simulink model "wheel_leg2"  (R2026a)
settings: Solver=VariableStepAuto  StopTime=7  MaxStep=0.01  AbsTol=1e-3  EnableMultiTasking=on
values from neighbouring files (symbols this model uses):
  K = lqr(A,B,Q,R)    [get_k_length.m]    (also in sys_lqr.m = sym('K',[2 6]))
  N = NM + mp*diff(x + L*sin(theta),t,2)    [get_k_length.m]
undefined symbols (not defined in the file or in its folder): X, Y, Z
libraries: sm_lib x87, nesl_utility x25, slpidlib x2
(part 1 of 3)
settings Model: Creator=86138  LastModifiedBy=Admin
settings SimscapeCC: SimscapeNominalValues="[{\"value\":\"1\",\"unit\":\"A\"},{\"value\":\"1\",\"unit\":\"bar\"},{\"value\":\"1\",\"unit\":\"cm^2\"},{\"value\":\"1\",\"unit\":\"cm^3/s\"},{\"value\":\"1\",\"unit\":\"kJ/kg\"},{\"value\":\"1\",\"unit\":\"kW\"},{\"value\":\"1\",\"unit\":\"l\"},{\"value\":\"1\",\"unit\":\"N\"},{\"value\":\"1\",\"unit\":\"N*m\"},{\"value\":\"1\",\"unit\":\"V\"}]"  SimscapeLogType=none  SimscapeLogSimulationStatistics=on
settings ExplorerConfigSet: InternalSimMechanicsExplorerSettings=|
  | <ExplorerConfiguration>
  | 
  |   <canonicalview>default</canonicalview>
  | 
  |   <TilePanel>
  |     <TileInfo>
  |       <Tiles Columns="1" Count="1" Height="898" Rows="1" Width="1720">
  |         <Row Weight="1"/>
  |         <Column Weight="1"/>
  |         <Tile Height="1" Width="1" X="0" Y="0"/>
  |       </Tiles>
  |     </TileInfo>
  |     <SceneInfo>
  |       <SceneViewer>
  |         <IsThisViewStd>
  |           <IsStandardView>off</IsStandardView>
  |           <StandardViewName>Front</StandardViewName>
  |         </IsThisViewStd>
  |         <BGColor>
  |           <R>0.85098039215686272</R>
  |           <G>0.85098039215686272</G>
  |           <B>0.85098039215686272</B>
  |           <A>1</A>
  |         </BGColor>
  |         <Camera>
  |           <DoPerspective>off</DoPerspective>
  |           <Position>
  |             <X>-61.687647663357318</X>
  |             <Y>-61.31400923411438</Y>
  |             <Z>24.215421272004388</Z>
  |           </Position>
  |           <Center>
  |             <X>-3.3890592997604467</X>
  |             <Y>3.6476545182531481</Y>
  |             <Z>2.021907302035288</Z>
  |           </Center>
  |           <Up>
  |             <X>0.16916832642928142</X>
  |             <Y>0.17928169149316647</Y>
  |             <Z>0.96914403079648859</Z>
  |           </Up>
  |           <XLim>2.9859335756375818</XLim>
  |           <YLim>2.9859335756375818</YLim>
  |           <ViewLimDist>0.01</ViewLimDist>
  |         </Camera>
  |       </SceneViewer>
  |     </SceneInfo>
  |   </TilePanel>
  | 
  |   <MechEditorPanel>
  |     <GfxPanelCameraMap/>
  |     <Cameras/>
  |     <VideoCreator>
  |       <IncludeTiles>All</IncludeTiles>
  |       <IncludeTime>on</IncludeTime>
  |       <IncludeWorldFrame>off</IncludeWorldFrame>
  |       <PlaybackSpeedRatio>0.5</PlaybackSpeedRatio>
  |       <FrameRate>30</FrameRate>
  |       <FrameSize>auto</FrameSize>
  |       <VideoFormat>MotionJPEGAVI</VideoFormat>
  |     </VideoCreator>
  |   </MechEditorPanel>
  | 
  |   <PlaybackSettings>
  |     <PlaybackSpeedFactor>0.5</PlaybackSpeedFactor>
  |   </PlaybackSettings>
  | 
  | </ExplorerConfiguration>

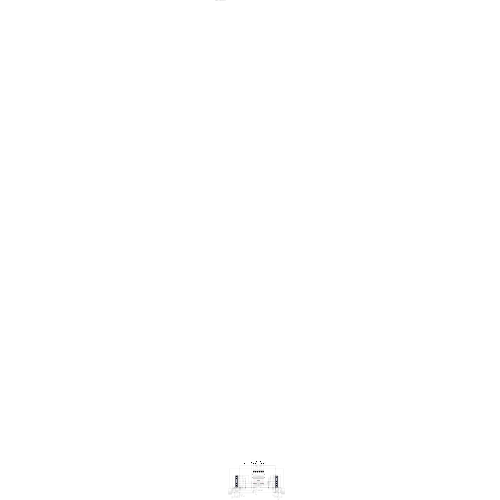
[thumbnail: Simulink's stored preview of the top-level diagram]
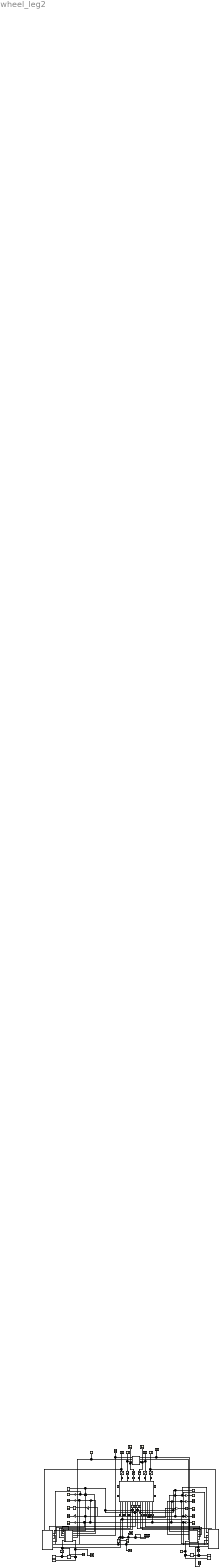
== system wheel_leg2 ==
  note: 参考开源文档作者：韭菜的菜 链接：https://zhuanlan.zhihu.com/p/613007726 来源：知乎
  note: K = get_k_length(0.25)
  Constant : Constant  Value=0.25
  Constant1 : Constant  Value=0.25
  Constant10 : Constant  Value=pi/2
  Constant12 : Constant  Value=pi/2
  Gain{22,24..26,33,36,38,40} (8 alike) : Gain  Gain=180/pi
  Gain29 : Gain  Gain=-0.06
  Gain41 : Gain  Gain=-0.06
  Integrator : Integrator
  Integrator2 : Integrator
  Integrator4 : Integrator
  L_X : Scope
      settings: ActiveDisplayYMinimum=-0.79846  ActiveDisplayYMaximum=7.01473
  L_d_phi : Scope
      settings: ActiveDisplayYMinimum=-7.35816  ActiveDisplayYMaximum=0.81757  DataLoggingVariableName=ScopeData2
  L_d_theta : Scope
      settings: ActiveDisplayYMinimum=-51.86845  ActiveDisplayYMaximum=175.83384  DataLoggingVariableName=ScopeData3
  L_phi : Scope
      settings: ActiveDisplayYMinimum=-1.27659  ActiveDisplayYMaximum=11.48927  DataLoggingVariableName=ScopeData4
  L_theta : Scope
      settings: ActiveDisplayYMinimum=-28.162  ActiveDisplayYMaximum=27.88738  DataLoggingVariableName=ScopeData5
  PID Controller2 : slpidlib/PID Controller  Controller=PID  Form=Parallel  TimeDomain=Continuous-time  UseExternalTs=off  SampleTime=-1  IntegratorMethod=Forward Euler  FilterMethod=Forward Euler  ControllerParametersSource=internal  P=500  I=0  UseKiTs=off  D=50  UseExternalDerivativeSource=off  N=100  UseFilter=on  TunerSelectOption=Transfer Function Based (PID Tuner App)  InitialConditionSource=internal  InitialConditionForIntegrator=0  InitialConditionForFilter=0  DifferentiatorICPrevScaledInput=0  ExternalReset=none  TrackingMode=off  Kt=1  LimitOutput=off  SatLimitsSource=internal  UpperSaturationLimit=inf  LowerSaturationLimit=-inf  LinearizeAsGain=on  AntiWindupMode=none  Kb=1  LimitIntegrator=off  UpperIntegratorSaturationLimit=inf  LowerIntegratorSaturationLimit=-inf  POutMin=[]  POutMax=[]  IOutMin=[]  IOutMax=[]  DOutMin=[]  DOutMax=[]  NOutMin=[]  NOutMax=[]  SumOutMin=[]  SumOutMax=[]  SaturationOutMin=[]  SaturationOutMax=[]  PParamMin=[]  PParamMax=[]  IParamMin=[]  IParamMax=[]  DParamMin=[]  DParamMax=[]  NParamMin=[]  NParamMax=[]  KbParamMin=[]  KbParamMax=[]  KtParamMin=[]  KtParamMax=[]  KbOutMin=[]  KbOutMax=[]  KtOutMin=[]  KtOutMax=[]  IntegratorOutMin=[]  IntegratorOutMax=[]  FilterOutMin=[]  FilterOutMax=[]  SumI1OutMin=[]  SumI1OutMax=[]  SumI2OutMin=[]  SumI2OutMax=[]  SumI3OutMin=[]  SumI3OutMax=[]  SumI4OutMin=[]  SumI4OutMax=[]  SumDOutMin=[]  SumDOutMax=[]  DifferentiatorOutMin=[]  DifferentiatorOutMax=[]  FilterDiffOutCoefMin=[]  FilterDiffOutCoefMax=[]  ReciprocalOutMin=[]  ReciprocalOutMax=[]  SumDenOutMin=[]  SumDenOutMax=[]  SumNumOutMin=[]  SumNumOutMax=[]  DivideOutMin=[]  DivideOutMax=[]  UdiffTsProdOutMin=[]  UdiffTsProdOutMax=[]  NTsProdOutMin=[]  NTsProdOutMax=[]  UintegralTsProdOutMin=[]  UintegralTsProdOutMax=[]  UngainTsProdOutMin=[]  UngainTsProdOutMax=[]  ClampingZeroOutDataTypeStr=Inherit: Inherit via back propagation  ClampingZeroOutMin=[]  ClampingZeroOutMax=[]  FilterDenConstantOutDataTypeStr=Inherit: Inherit via back propagation  FilterDenConstantOutMin=[]  FilterDenConstantOutMax=[]  PCopyOutDataTypeStr=Inherit: Inherit via back propagation  PCopyOutMin=[]  PCopyOutMax=[]  NCopyOutDataTypeStr=Inherit: Inherit via back propagation  NCopyOutMin=[]  NCopyOutMax=[]  IntegratorContinuousStateAttributes=''  IntegratorStateMustResolveToSignalObject=off  IntegratorRTWStateStorageClass=Auto  FilterContinuousStateAttributes=''  FilterStateMustResolveToSignalObject=off  FilterRTWStateStorageClass=Auto  ParallelPVariant=InternalParameters  IdealPVariant=Disabled  IVariant=InternalParameters  DVariant=InternalParameters  IntegratorVariant=Continuous  SatVariant=Disabled  AWVariant=Passthrough  PCopyVariant=Disabled  TRVariant=Disabled  FdbkBlocksVariant=Forward  IdealPFdbkVariant=Disabled  SatFdbkVariant=Disabled  DerivativeFilterVariant=ContFilter  NVariant=InternalParameters  NCopyVariant=Disabled  FilterICVariant=InternalICsFilter  IntegratorICVariant=InternalICs  ExternalResetVariant=Disabled  TRSumVariant=Passthrough  SumFdbkVariant=Disabled  SumVariant=Sum_PID  TsampFilterVariant=InternalTs  TsampNgainVariant=Passthrough  TsampIntegralVariant=Disabled_SignalSpec  ExternalSaturationOutDataTypeStr=Inherit: Same as second input  DerivativeSourceVariant=ErrorSignal  PreIntVariant=InternalPreInt
  PID Controller3 : slpidlib/PID Controller  Controller=PID  Form=Parallel  TimeDomain=Continuous-time  UseExternalTs=off  SampleTime=-1  IntegratorMethod=Forward Euler  FilterMethod=Forward Euler  ControllerParametersSource=internal  P=500  I=0  UseKiTs=off  D=50  UseExternalDerivativeSource=off  N=100  UseFilter=on  TunerSelectOption=Transfer Function Based (PID Tuner App)  InitialConditionSource=internal  InitialConditionForIntegrator=0  InitialConditionForFilter=0  DifferentiatorICPrevScaledInput=0  ExternalReset=none  TrackingMode=off  Kt=1  LimitOutput=off  SatLimitsSource=internal  UpperSaturationLimit=inf  LowerSaturationLimit=-inf  LinearizeAsGain=on  AntiWindupMode=none  Kb=1  LimitIntegrator=off  UpperIntegratorSaturationLimit=inf  LowerIntegratorSaturationLimit=-inf  POutMin=[]  POutMax=[]  IOutMin=[]  IOutMax=[]  DOutMin=[]  DOutMax=[]  NOutMin=[]  NOutMax=[]  SumOutMin=[]  SumOutMax=[]  SaturationOutMin=[]  SaturationOutMax=[]  PParamMin=[]  PParamMax=[]  IParamMin=[]  IParamMax=[]  DParamMin=[]  DParamMax=[]  NParamMin=[]  NParamMax=[]  KbParamMin=[]  KbParamMax=[]  KtParamMin=[]  KtParamMax=[]  KbOutMin=[]  KbOutMax=[]  KtOutMin=[]  KtOutMax=[]  IntegratorOutMin=[]  IntegratorOutMax=[]  FilterOutMin=[]  FilterOutMax=[]  SumI1OutMin=[]  SumI1OutMax=[]  SumI2OutMin=[]  SumI2OutMax=[]  SumI3OutMin=[]  SumI3OutMax=[]  SumI4OutMin=[]  SumI4OutMax=[]  SumDOutMin=[]  SumDOutMax=[]  DifferentiatorOutMin=[]  DifferentiatorOutMax=[]  FilterDiffOutCoefMin=[]  FilterDiffOutCoefMax=[]  ReciprocalOutMin=[]  ReciprocalOutMax=[]  SumDenOutMin=[]  SumDenOutMax=[]  SumNumOutMin=[]  SumNumOutMax=[]  DivideOutMin=[]  DivideOutMax=[]  UdiffTsProdOutMin=[]  UdiffTsProdOutMax=[]  NTsProdOutMin=[]  NTsProdOutMax=[]  UintegralTsProdOutMin=[]  UintegralTsProdOutMax=[]  UngainTsProdOutMin=[]  UngainTsProdOutMax=[]  ClampingZeroOutDataTypeStr=Inherit: Inherit via back propagation  ClampingZeroOutMin=[]  ClampingZeroOutMax=[]  FilterDenConstantOutDataTypeStr=Inherit: Inherit via back propagation  FilterDenConstantOutMin=[]  FilterDenConstantOutMax=[]  PCopyOutDataTypeStr=Inherit: Inherit via back propagation  PCopyOutMin=[]  PCopyOutMax=[]  NCopyOutDataTypeStr=Inherit: Inherit via back propagation  NCopyOutMin=[]  NCopyOutMax=[]  IntegratorContinuousStateAttributes=''  IntegratorStateMustResolveToSignalObject=off  IntegratorRTWStateStorageClass=Auto  FilterContinuousStateAttributes=''  FilterStateMustResolveToSignalObject=off  FilterRTWStateStorageClass=Auto  ParallelPVariant=InternalParameters  IdealPVariant=Disabled  IVariant=InternalParameters  DVariant=InternalParameters  IntegratorVariant=Continuous  SatVariant=Disabled  AWVariant=Passthrough  PCopyVariant=Disabled  TRVariant=Disabled  FdbkBlocksVariant=Forward  IdealPFdbkVariant=Disabled  SatFdbkVariant=Disabled  DerivativeFilterVariant=ContFilter  NVariant=InternalParameters  NCopyVariant=Disabled  FilterICVariant=InternalICsFilter  IntegratorICVariant=InternalICs  ExternalResetVariant=Disabled  TRSumVariant=Passthrough  SumFdbkVariant=Disabled  SumVariant=Sum_PID  TsampFilterVariant=InternalTs  TsampNgainVariant=Passthrough  TsampIntegralVariant=Disabled_SignalSpec  ExternalSaturationOutDataTypeStr=Inherit: Same as second input  DerivativeSourceVariant=ErrorSignal  PreIntVariant=InternalPreInt
  PS-Simulink Converter{18..24,27..37} (18 alike) : nesl_utility/PS-Simulink Converter  PhysicalDomain=network_engine_domain  SubClassName=ps_output  LeftPortType=input  RightPortType=output  PseudoPeriodic=off  Frequencies=[]  VectorFormat=1-D array  Unit=inherit  AffineConversion=off
  R_X : Scope
      settings: ActiveDisplayYMinimum=-0.7616  ActiveDisplayYMaximum=6.68295  DataLoggingVariableName=ScopeData6
  R_d_phi : Scope
      settings: ActiveDisplayYMinimum=-7.35816  ActiveDisplayYMaximum=0.81757  DataLoggingVariableName=ScopeData7
  R_d_theta : Scope
      settings: ActiveDisplayYMinimum=-391.81986  ActiveDisplayYMaximum=622.66027  DataLoggingVariableName=ScopeData8
  R_phi : Scope
      settings: ActiveDisplayYMinimum=-1.27659  ActiveDisplayYMaximum=11.48927  DataLoggingVariableName=ScopeData9
  R_theta : Scope
      settings: ActiveDisplayYMinimum=-1.24478  ActiveDisplayYMaximum=0.73055  DataLoggingVariableName=ScopeData10
  Saturation{1..4} (4 alike) : Saturate  UpperLimit=100  LowerLimit=-100
  Saturation5 : Saturate  UpperLimit=300  LowerLimit=-300
  Saturation6 : Saturate  UpperLimit=300  LowerLimit=-300
  Saturation7 : Saturate  UpperLimit=9  LowerLimit=-9
  Saturation8 : Saturate  UpperLimit=9  LowerLimit=-9
  Scope{,1..15} (16 alike) : Scope
      Scope settings: ActiveDisplayYMinimum=0.07562  ActiveDisplayYMaximum=0.4295  DataLoggingVariableName=ScopeData11
      Scope1 settings: ActiveDisplayYMinimum=-9.10613  ActiveDisplayYMaximum=7.92497  DataLoggingVariableName=ScopeData12
      Scope10 settings: ActiveDisplayYMinimum=-375  ActiveDisplayYMaximum=375  DataLoggingVariableName=ScopeData20
      Scope11 settings: ActiveDisplayYMinimum=-1  ActiveDisplayYMaximum=1  DataLoggingVariableName=ScopeData21
      Scope12 settings: ActiveDisplayYMinimum=0.07562  ActiveDisplayYMaximum=0.4295  DataLoggingVariableName=ScopeData22
      Scope13 settings: ActiveDisplayYMinimum=-3.1177392671437287  ActiveDisplayYMaximum=3.1442797487223748
      Scope14 settings: ActiveDisplayYMinimum=-0.31249999999999994  ActiveDisplayYMaximum=2.8125  DataLoggingVariableName=ScopeData2
      Scope15 settings: ActiveDisplayYMinimum=-3.2783000855407103  ActiveDisplayYMaximum=0.36501807360702582  DataLoggingVariableName=ScopeData3
      Scope2 settings: ActiveDisplayYMinimum=-47.6537  ActiveDisplayYMaximum=22.13517  DataLoggingVariableName=ScopeData13
      Scope3 settings: ActiveDisplayYMinimum=-22.13977  ActiveDisplayYMaximum=47.6548  DataLoggingVariableName=ScopeData14
      Scope4 settings: ActiveDisplayYMinimum=-22.14008  ActiveDisplayYMaximum=47.65761  DataLoggingVariableName=ScopeData15
      Scope5 settings: ActiveDisplayYMinimum=-47.65142  ActiveDisplayYMaximum=22.13492  DataLoggingVariableName=ScopeData16
      Scope6 settings: ActiveDisplayYMinimum=-18.05595  ActiveDisplayYMaximum=36.45588
      Scope7 settings: ActiveDisplayYMinimum=-39.05246  ActiveDisplayYMaximum=39.58723  DataLoggingVariableName=ScopeData17
      Scope8 settings: ActiveDisplayYMinimum=-39.6576  ActiveDisplayYMaximum=39.74338  DataLoggingVariableName=ScopeData18
      Scope9 settings: ActiveDisplayYMinimum=-212.85082  ActiveDisplayYMaximum=356.98342  DataLoggingVariableName=ScopeData19
  Simulink-PS Converter{1..6} (6 alike) : nesl_utility/Simulink-PS Converter  PhysicalDomain=network_engine_domain  SubClassName=ps_input  LeftPortType=input  RightPortType=output  PseudoPeriodic=off  Frequencies=[]  NoiseDistribution=none  NoiseParameters=[]  Unit=1  AffineConversion=off  FilteringAndDerivatives=provide  SimscapeFilterOrder=1  InputFilterTimeConstant=0.001  UdotUserProvided=0
  Step2 : Step  Time=0.2  FinalValue=2.5  SampleTime=0
  Step3 : Step  Time=7  FinalValue=2.5  SampleTime=0
  Subsystem1 : Subsystem
      settings: PortSchema="{\"entries\":[{\"content\":{\"sides\":[{\"content\":{\"connectorIds\":[\"In1\",\"In2\",\"In3\",\"In4\",\"In5\",\"In6\"]},\"type\":\"ConnectorPlacement.EquallySpacedRectSide\",\"uuid\":\"055cb80c-cd03-4a8d-aef8-6b3df8c72d3f\"},{\"content\":{\"connectorIds\":[],\"side\":\"RIGHT\"},\"type\":\"ConnectorPlacement.EquallySpacedRectSide\",\"uuid\":\"5756fad1-d70f-4a11-a5af-d2f67bfb0d7e\"},{\"content\":{\"connectorIds\":[\"Out1\",\"Out2\"],\"side\":\"TOP\"},\"type\":\"ConnectorPlacement.EquallySpacedRectSide\",\"uuid\":\"9c70cf42-10f8-4525-9406-562484abf580\"}]},\"type\":\"ConnectorPlacement.EquallySpacedConnector\",\"uuid\":\"7084d402-0e44-4d2f-8cc2-1336d196e84d\"}],\"packageUris\":[\"http://schema.mathworks.com/mf0/Connector/R2020b\"],\"version\":\"1.0\"}"
  Subsystem4 : Subsystem
      settings: PortSchema="{\"entries\":[{\"content\":{\"sides\":[{\"content\":{\"connectorIds\":[\"In1\",\"In2\",\"In3\",\"In4\",\"In5\"]},\"type\":\"ConnectorPlacement.EquallySpacedRectSide\",\"uuid\":\"40de31e0-cc19-460f-99e9-affbb47f7204\"},{\"content\":{\"connectorIds\":[\"Out1\",\"Out2\",\"Out3\",\"Out4\",\"Out5\"],\"side\":\"RIGHT\"},\"type\":\"ConnectorPlacement.EquallySpacedRectSide\",\"uuid\":\"e61df4ab-633d-456a-aa2d-223df880274d\"},{\"content\":{\"connectorIds\":[\"In6\"],\"side\":\"TOP\"},\"type\":\"ConnectorPlacement.EquallySpacedRectSide\",\"uuid\":\"a7334146-3144-4ab1-9f08-8bf1583597b4\"}]},\"type\":\"ConnectorPlacement.EquallySpacedConnector\",\"uuid\":\"1490fe93-b025-4c86-96e6-b1bfc13c7f50\"}],\"packageUris\":[\"http://schema.mathworks.com/mf0/Connector/R2020b\"],\"version\":\"1.0\"}"
  Sum13 : Sum  Inputs=++|
  Sum14 : Sum  Inputs=|++
  Sum15 : Sum  Inputs=|++
  Sum16 : Sum  Inputs=|--
  Sum17 : Sum  Inputs=+--
  Sum18 : Sum  Inputs=+|+
  Sum20 : Sum  Inputs=++|
  Sum22 : Sum  Inputs=+-|
  Sum23 : Sum  Inputs=-|+
  Sum24 : Sum  Inputs=+--
  Sum25 : Sum  Inputs=+|+
  Sum26 : Sum  Inputs=+-|
  Sum27 : Sum  Inputs=|--
  Sum29 : Sum  Inputs=-|+
  blance_leg_model : Subsystem
      settings: PortSchema="{\"entries\":[{\"content\":{\"sides\":[{\"content\":{\"connectorIds\":[\"LConn1\",\"LConn2\",\"LConn3\",\"LConn4\",\"LConn5\",\"LConn6\"]},\"type\":\"ConnectorPlacement.EquallySpacedRectSide\",\"uuid\":\"df2d0b15-ec70-4430-8d90-67c6d88950b4\"},{\"content\":{\"connectorIds\":[\"RConn1\",\"RConn2\",\"RConn3\",\"RConn4\",\"RConn5\",\"RConn6\",\"RConn7\",\"RConn8\",\"RConn9\",\"RConn10\",\"RConn11\",\"RConn12\",\"RConn13\",\"RConn14\"],\"side\":\"RIGHT\"},\"type\":\"ConnectorPlacement.EquallySpacedRectSide\",\"uuid\":\"ec9b4787-d265-4ad9-b676-e253d2304993\"},{\"content\":{\"connectorIds\":[\"LConn7\",\"LConn8\"],\"side\":\"TOP\"},\"type\":\"ConnectorPlacement.EquallySpacedRectSide\",\"uuid\":\"40dd08fe-dc32-4cee-bbb8-c1ec6d04ee32\"},{\"content\":{\"connectorIds\":[\"RConn15\",\"RConn16\"],\"side\":\"BOTTOM\"},\"type\":\"ConnectorPlacement.EquallySpacedRectSide\",\"uuid\":\"0f9c1faf-3e52-4dca-bbb1-0993be9fa88c\"}]},\"type\":\"ConnectorPlacement.EquallySpacedConnector\",\"uuid\":\"d540d646-85aa-4f97-ae4d-1bccec971368\"}],\"packageUris\":[\"http://schema.mathworks.com/mf0/Connector/R2020b\"],\"version\":\"1.0\"}"
  calc : Subsystem
      settings: PortSchema="{\"entries\":[{\"content\":{\"sides\":[{\"content\":{\"connectorIds\":[\"In1\",\"In2\",\"In3\",\"In4\",\"In5\",\"In6\"]},\"type\":\"ConnectorPlacement.EquallySpacedRectSide\",\"uuid\":\"055cb80c-cd03-4a8d-aef8-6b3df8c72d3f\"},{\"content\":{\"connectorIds\":[],\"side\":\"RIGHT\"},\"type\":\"ConnectorPlacement.EquallySpacedRectSide\",\"uuid\":\"5756fad1-d70f-4a11-a5af-d2f67bfb0d7e\"},{\"content\":{\"connectorIds\":[\"Out1\",\"Out2\"],\"side\":\"TOP\"},\"type\":\"ConnectorPlacement.EquallySpacedRectSide\",\"uuid\":\"9c70cf42-10f8-4525-9406-562484abf580\"}]},\"type\":\"ConnectorPlacement.EquallySpacedConnector\",\"uuid\":\"7084d402-0e44-4d2f-8cc2-1336d196e84d\"}],\"packageUris\":[\"http://schema.mathworks.com/mf0/Connector/R2020b\"],\"version\":\"1.0\"}"
  control : Subsystem
      settings: PortSchema="{\"entries\":[{\"content\":{\"sides\":[{\"content\":{\"connectorIds\":[\"In1\",\"In2\",\"In3\",\"In4\",\"In5\"]},\"type\":\"ConnectorPlacement.EquallySpacedRectSide\",\"uuid\":\"40de31e0-cc19-460f-99e9-affbb47f7204\"},{\"content\":{\"connectorIds\":[\"Out1\",\"Out2\",\"Out3\",\"Out4\",\"Out5\"],\"side\":\"RIGHT\"},\"type\":\"ConnectorPlacement.EquallySpacedRectSide\",\"uuid\":\"e61df4ab-633d-456a-aa2d-223df880274d\"},{\"content\":{\"connectorIds\":[\"In6\"],\"side\":\"TOP\"},\"type\":\"ConnectorPlacement.EquallySpacedRectSide\",\"uuid\":\"a7334146-3144-4ab1-9f08-8bf1583597b4\"}]},\"type\":\"ConnectorPlacement.EquallySpacedConnector\",\"uuid\":\"1490fe93-b025-4c86-96e6-b1bfc13c7f50\"}],\"packageUris\":[\"http://schema.mathworks.com/mf0/Connector/R2020b\"],\"version\":\"1.0\"}"
  jump_control : Subsystem  mask{jump_time=3.5}
      mask prompts: jump_time "跳跃时间"
      settings: PortSchema="{\"entries\":[{\"content\":{\"sides\":[{\"content\":{\"connectorIds\":[\"In1\",\"In2\",\"Out3\",\"Out4\"]},\"type\":\"ConnectorPlacement.EquallySpacedRectSide\",\"uuid\":\"555f1eec-a1f8-4438-898b-242296387de2\"},{\"content\":{\"connectorIds\":[\"In3\",\"In4\",\"Out1\",\"Out2\"],\"side\":\"RIGHT\"},\"type\":\"ConnectorPlacement.EquallySpacedRectSide\",\"uuid\":\"4e34be98-beb2-4e32-b120-d99682746887\"},{\"content\":{\"connectorIds\":[],\"side\":\"TOP\"},\"type\":\"ConnectorPlacement.EquallySpacedRectSide\",\"uuid\":\"2dbe6b4e-143a-4ee5-b634-fdf47ce3ae58\"}]},\"type\":\"ConnectorPlacement.EquallySpacedConnector\",\"uuid\":\"fd4bce8e-8918-4201-9e0d-25b1dfe9d9e9\"}],\"packageUris\":[\"http://schema.mathworks.com/mf0/Connector/R2020b\"],\"version\":\"1.0\"}"
      mask DialogControl ParameterGroupVar Prompt: 参数
  除去轮子后机体重量 : Constant  Value=62.5
  除去轮子后机体重量， : Constant  Value=62.5
  wires:
  Integrator4/1 -> L_X/1  "x"
  Saturation8/1 -> Simulink-PS Converter4/1
  Saturation7/1 -> Simulink-PS Converter6/1
  Constant10/1 -> Sum20/1, Sum13/1, Sum24/1
  Subsystem4/5(L0) -> Sum29/1, Scope/1
  Subsystem1/2(T) -> Saturation8/1, Scope6/1
  Sum23/1 -> PID Controller2/1
  Subsystem4/3(T1) -> jump_control/3(L_Tp1_in), Scope7/1
  PS-Simulink Converter34/1 -> Sum20/2
  Sum22/1 -> Scope14/1, Sum26/2  "speed_set"
  Saturation5/1 -> Scope10/1, Subsystem4/5(F0)
  calc/2(T) -> Saturation7/1, Scope1/1
  Gain25/1 -> L_d_theta/1
  Integrator/1 -> Scope15/1, Subsystem1/5(x), calc/5(x)
  Gain41/1 -> Integrator2/1  "x'"
  jump_control/4(R_Tp4) -> Scope3/1, Saturation2/1
  PS-Simulink Converter33/1 -> Sum14/1
  Sum26/1 -> Scope13/1, Integrator/1
  control/4(T2) -> jump_control/2(R_Tp2_in), Scope11/1
  Saturation6/1 -> Scope9/1, control/5(F0)
  Subsystem4/4(T2) -> jump_control/4(L_Tp2_in)
  Gain26/1 -> L_d_phi/1
  jump_control/2(L_Tp4) -> Scope4/1, Saturation3/1
  Constant1/1 -> Sum23/2
  Sum18/1 -> Saturation5/1
  Sum15/1 -> Subsystem4/2(phi4)
  Sum25/1 -> Saturation6/1
  Gain36/1 -> R_theta/1
  Sum27/1 -> Subsystem1/2(d_theta), Gain25/1
  Subsystem4/2(d_phi0) -> Sum27/1
  PS-Simulink Converter32/1 -> Sum13/2
  calc/1(Tp) -> control/6(Tp)
  Constant12/1 -> Sum15/2, Sum14/2, Sum17/1
  control/2(d_phi0) -> Sum16/1
  Sum17/1 -> Subsystem1/1(theta), Gain24/1
  control/5(L0) -> Scope12/1, Sum23/1
  PS-Simulink Converter19/1 -> calc/6(d_x), Subsystem1/6(d_x), Sum26/1
  PS-Simulink Converter29/1 -> control/4(d_phi4)
  PS-Simulink Converter24/1 -> calc/4(d_phi), Gain40/1, Sum16/2, Subsystem1/4(d_phi), Gain26/1, Sum27/2
  PS-Simulink Converter23/1 -> calc/3(phi), Gain22/1, Sum24/3, Subsystem1/3(phi), Gain33/1, Sum17/3
  Gain29/1 -> Integrator4/1  "x'"
  PS-Simulink Converter31/1 -> control/3(d_phi1)
  Sum14/1 -> Subsystem4/1(phi1)
  Sum13/1 -> control/1(phi1)
  jump_control/1(L_Tp1) -> Saturation4/1, Scope5/1
  PS-Simulink Converter20/1 -> Subsystem4/3(d_phi1)
  PS-Simulink Converter22/1 -> Gain29/1
  Integrator2/1 -> R_X/1  "x"
  PS-Simulink Converter21/1 -> Subsystem4/4(d_phi4)
  PS-Simulink Converter28/1 -> Gain41/1
  control/3(T1) -> Scope8/1, jump_control/1(R_Tp1_in)
  Saturation2/1 -> Simulink-PS Converter3/1
  Sum20/1 -> control/2(phi4)
  除去轮子后机体重量/1 -> Sum18/2
  control/1(phi0) -> Sum24/2
  Gain38/1 -> R_d_theta/1
  PS-Simulink Converter35/1 -> Sum15/1
  Saturation4/1 -> Simulink-PS Converter5/1
  jump_control/3(R_Tp1) -> Saturation1/1, Scope2/1
  Sum24/1 -> calc/1(theta), Gain36/1
  PID Controller3/1 -> Sum18/1
  Saturation3/1 -> Simulink-PS Converter2/1
  Gain33/1 -> L_phi/1
  Gain24/1 -> L_theta/1
  Sum16/1 -> calc/2(d_theta), Gain38/1
  Constant/1 -> Sum29/2
  Sum29/1 -> PID Controller3/1
  Gain22/1 -> R_phi/1
  Saturation1/1 -> Simulink-PS Converter1/1
  Gain40/1 -> R_d_phi/1
  Subsystem4/1(phi0) -> Sum17/2
  除去轮子后机体重量，/1 -> Sum25/1
  PID Controller2/1 -> Sum25/2
  Subsystem1/1(Tp) -> Subsystem4/6(Tp)
  Step2/1 -> Sum22/1
  Step3/1 -> Sum22/2
  connections:
  PS-Simulink Converter28/LConn1 -- blance_leg_model/RConn3
  PS-Simulink Converter35/LConn1 -- blance_leg_model/RConn9
  PS-Simulink Converter29/LConn1 -- blance_leg_model/RConn4
  PS-Simulink Converter33/LConn1 -- blance_leg_model/RConn8
  PS-Simulink Converter31/LConn1 -- blance_leg_model/RConn5
  Simulink-PS Converter6/RConn1 -- blance_leg_model/LConn1
  PS-Simulink Converter36/LConn1 -- blance_leg_model/RConn15
  PS-Simulink Converter30/LConn1 -- blance_leg_model/LConn8
  Simulink-PS Converter3/RConn1 -- blance_leg_model/LConn3
  PS-Simulink Converter27/LConn1 -- blance_leg_model/LConn7
  PS-Simulink Converter24/LConn1 -- blance_leg_model/RConn14
  PS-Simulink Converter22/LConn1 -- blance_leg_model/RConn12
  PS-Simulink Converter21/LConn1 -- blance_leg_model/RConn11
  Simulink-PS Converter2/RConn1 -- blance_leg_model/LConn4
  PS-Simulink Converter20/LConn1 -- blance_leg_model/RConn10
  PS-Simulink Converter23/LConn1 -- blance_leg_model/RConn13
  PS-Simulink Converter19/LConn1 -- blance_leg_model/RConn2
  PS-Simulink Converter37/LConn1 -- blance_leg_model/RConn16
  Simulink-PS Converter5/RConn1 -- blance_leg_model/LConn5
  PS-Simulink Converter18/LConn1 -- blance_leg_model/RConn1
  PS-Simulink Converter32/LConn1 -- blance_leg_model/RConn6
  Simulink-PS Converter1/RConn1 -- blance_leg_model/LConn2
  PS-Simulink Converter34/LConn1 -- blance_leg_model/RConn7
  Simulink-PS Converter4/RConn1 -- blance_leg_model/LConn6

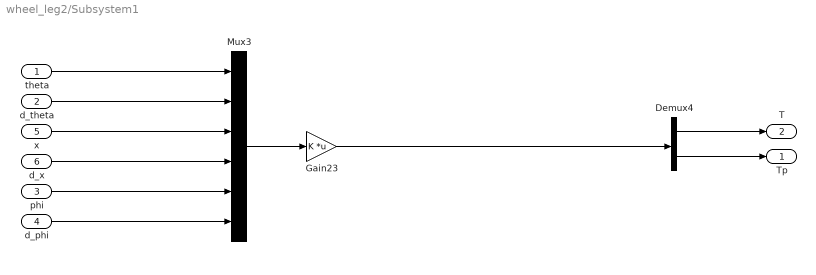
== system wheel_leg2/Subsystem1 ==
  theta : Inport
  d_theta : Inport  Port=2
  phi : Inport  Port=3
  d_phi : Inport  Port=4
  x : Inport  Port=5
  d_x : Inport  Port=6
  Demux4 : Demux  Outputs=2
  Gain23 : Gain  Gain=K  Multiplication=Matrix(K*u) (u vector)
  Mux3 : Mux  Inputs=6
  Tp : Outport
  T : Outport  Port=2
  wires:
  theta/1 -> Mux3/1
  d_theta/1 -> Mux3/2
  d_x/1 -> Mux3/4
  d_phi/1 -> Mux3/6
  phi/1 -> Mux3/5
  Demux4/2 -> Tp/1
  x/1 -> Mux3/3
  Mux3/1 -> Gain23/1
  Gain23/1 -> Demux4/1
  Demux4/1 -> T/1

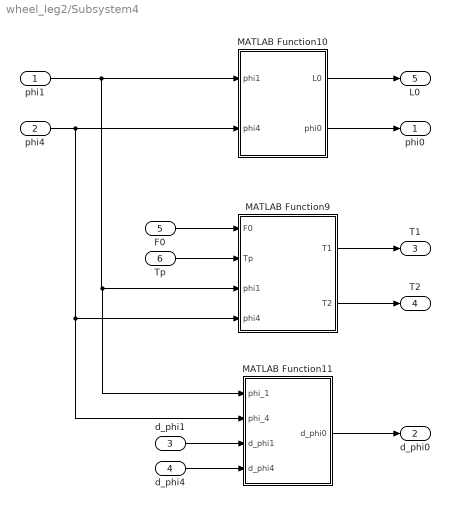
== system wheel_leg2/Subsystem4 ==
  phi1 : Inport
  phi4 : Inport  Port=2
  d_phi1 : Inport  Port=3
  d_phi4 : Inport  Port=4
  F0 : Inport  Port=5
  Tp : Inport  Port=6
  MATLAB Function10 : MATLAB Function  TreatAsAtomicUnit=on
  MATLAB Function11 : MATLAB Function  TreatAsAtomicUnit=on
  MATLAB Function9 : MATLAB Function  TreatAsAtomicUnit=on
  phi0 : Outport
  d_phi0 : Outport  Port=2
  T1 : Outport  Port=3
  T2 : Outport  Port=4
  L0 : Outport  Port=5
  wires:
  phi1/1 -> MATLAB Function11/1(phi_1), MATLAB Function9/3(phi1), MATLAB Function10/1(phi1)
  MATLAB Function10/2(phi0) -> phi0/1
  MATLAB Function11/1(d_phi0) -> d_phi0/1
  Tp/1 -> MATLAB Function9/2(Tp)
  d_phi4/1 -> MATLAB Function11/4(d_phi4)
  d_phi1/1 -> MATLAB Function11/3(d_phi1)
  MATLAB Function9/1(T1) -> T1/1
  phi4/1 -> MATLAB Function11/2(phi_4), MATLAB Function9/4(phi4), MATLAB Function10/2(phi4)
  F0/1 -> MATLAB Function9/1(F0)
  MATLAB Function9/2(T2) -> T2/1
  MATLAB Function10/1(L0) -> L0/1
